simulink model "SRLatchTest"  (R2016a)
settings: Solver=VariableStepAuto  StartTime=0.0  StopTime=1  RelTol=1e-3
libraries: SimscapeMacros x10, nesl_utility x5, ProjectBlocks x2
settings Model: Creator=Peter  LastModifiedBy=Peter

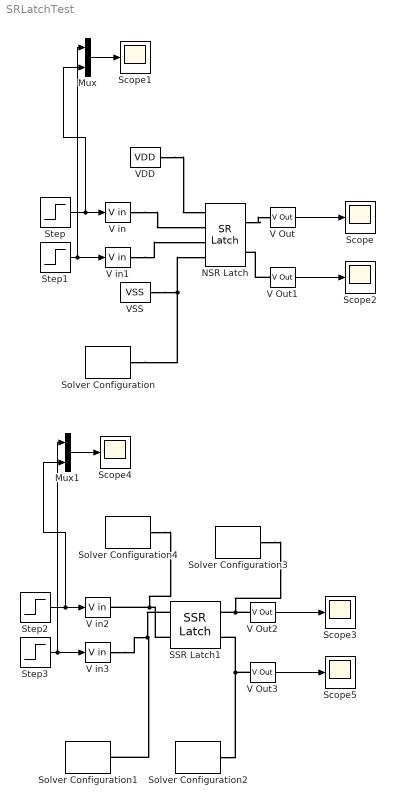
== system SRLatchTest ==
  Mux : Mux  Inputs=2
  Mux1 : Mux  Inputs=2
  NSR Latch : ProjectBlocks/SR Latch
  SSR Latch1 : ProjectBlocks/Axis Integrator Old/SSR Latch
  Scope{,1..5} (6 alike) : Scope
  Solver Configuration{,1..4} (5 alike) : nesl_utility/Solver Configuration  PhysicalDomain=network_engine_domain  SubClassName=solver  LeftPortType=input  RightPortType=generic  Accelerate=off  Tones=[]  Harmonics=[]  SimulateNoise=off  Profile=off  UseLocalSampling=off  EnableSwitchedLinearOptims=on  FrequencyDomain=off  UseCCode=off  RelTol=0.001  AbsTol=1e-06  MinStep=1e-09  ToWorkspace=off  RevertToSquareIcSolve=off  NumHomotopyIterations=100  PhasorMode=off  PhasorModeNumHarmonics=1  OverrideAbsTol=off  DoDC=off  ResidualTolerance=1e-09  UseLocalSolver=off  LocalSolverChoice=NE_BACKWARD_EULER_ADVANCER  LocalSolverSampleTime=0.001  DoFixedCost=off  MaxNonlinIter=3  MaxModeIter=2  LinearAlgebra=Sparse  DelaysMemoryBudget=1024  AutomaticFiltering=on  FilteringTimeConstant=0.001
  Step : Step  Time=.3  Before=-10  After=10  SampleTime=0
  Step1 : Step  Time=.7  Before=10  After=-10  SampleTime=0
  Step2 : Step  Time=.3  Before=-10  After=10  SampleTime=0
  Step3 : Step  Time=.7  Before=10  After=-10  SampleTime=0
  V Out{,1..3} (4 alike) : SimscapeMacros/V Out
  V in{,1..3} (4 alike) : SimscapeMacros/V in
  VDD : SimscapeMacros/VDD
  VSS : SimscapeMacros/VSS
  wires:
  V Out/1 -> Scope/1
  Step/1 -> Mux/2, V in/1
  Step1/1 -> Mux/1, V in1/1
  Mux/1 -> Scope1/1
  V Out1/1 -> Scope2/1
  V Out2/1 -> Scope3/1
  Step2/1 -> Mux1/2, V in2/1
  Step3/1 -> Mux1/1, V in3/1
  Mux1/1 -> Scope4/1
  V Out3/1 -> Scope5/1
  connections:
  VDD/RConn1 -- NSR Latch/LConn1
  VSS/RConn1 -- NSR Latch/LConn4 -- Solver Configuration/RConn1
  NSR Latch/RConn1 -- V Out/LConn1
  V Out1/LConn1 -- NSR Latch/RConn2
  V in/RConn1 -- NSR Latch/LConn2
  V in1/RConn1 -- NSR Latch/LConn3
  V Out2/LConn1 -- Solver Configuration3/RConn1 -- SSR Latch1/RConn1
  V Out3/LConn1 -- Solver Configuration2/RConn1 -- SSR Latch1/RConn2
  V in3/RConn1 -- SSR Latch1/LConn1 -- Solver Configuration1/RConn1
  SSR Latch1/LConn2 -- Solver Configuration4/RConn1 -- V in2/RConn1
